simulink model "DepthTracking_ALOS_ADRC"  (R2020b)
settings: Solver=ode1  StartTime=0.0  StopTime=80  FixedStep=0.1  RelTol=1e-3
InitFcn:
  | InitParam;
undefined symbols (not defined in the file or in its folder): sigbuilder_block
settings Model: Creator=53549  LastModifiedBy=53549
settings DataIOCC: ReturnWorkspaceOutputs=off
settings DebuggingCC: ArithmeticOperatorsInVariantConditions=warning
settings SFSimCC: SimUseLocalCustomCode=off  CustomCodeUndefinedFunction=UseInterfaceOnly
settings RTWCC: RTWUseLocalCustomCode=off
settings CodeAppCC: StateflowObjectComments=on

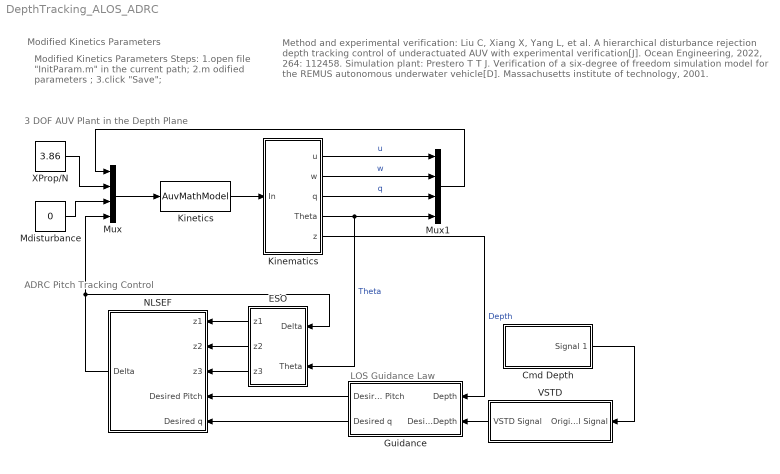
== system DepthTracking_ALOS_ADRC ==
  note: LOS Guidance Law
  note: ADRC Pitch Tracking Control
  note: 3 DOF AUV Plant in the Depth Plane
  note: Method and experimental verification: Liu C, Xiang X, Yang L, et al. A hierarchical disturbance rejection depth tracking control of underactuated AUV with experimental verification[J]. Ocean Engineering, 2022, 264: 112458.
      | Simulation plant: Prestero T T J. Verification of a six-degree of freedom simulation model for the REMUS autonomous underwater vehicle[D]. Massachusetts institute of technology, 2001.
  note: Modified Kinetics Parameters Steps:
      | 1.open file "InitParam.m" in the current path;
      | 2.m odified parameters ;
      | 3.click "Save";
  note: Modified Kinetics Parameters
  Cmd Depth : Subsystem  Tag=STV Subsys  LoadFcn=sigbuilder_block('load');  StartFcn=sigbuilder_block('start');  StopFcn=sigbuilder_block('stop');  ClipboardFcn=sigbuilder_block('clipboard');  mask(Sigbuilder block){tuvar=[0:10]}
      mask help: Simulink:masks:SigbuilderBlock_MD
      mask init:
      | if ~strcmp(get_param(bdroot(gcbh),'SimulationStatus'),'stopped') tuvar = sigbuilder_block('maskInit'); end
      settings: CopyFcn=sigbuilder_block('copy');  DeleteFcn=sigbuilder_block('delete');  ModelCloseFcn=sigbuilder_block('modelClose');  PreSaveFcn=sigbuilder_block('preSave');  PauseFcn=sigbuilder_block('pause');  ContinueFcn=sigbuilder_block('continue');  NameChangeFcn=sigbuilder_block('namechange');  OpenFcn=sigbuilder_block('open',[75 86 550.5 363 ]);  CloseFcn=sigbuilder_block('close');
      mask Display: plot(0, 0, 100, 100,[2, 2, 32, 32, 2], [68, 8, 8, 68, 68],[32, 2], [38, 38], [32, 19, 2],[53, 60, 44], [32, 17, 17, 2],[16, 16, 31, 31]);txt = getActiveGroup(gcbh);text(2, 100, txt,'verticalAlignment', 'top');
  ESO : Subsystem
  Guidance : Subsystem  mask{losAlg=ALOS, klos=3, KIlos=0.01}
      mask prompts: losAlg "LOS Form"; klos "Forward Distance"; KIlos "Integral gain"
      mask TypeOptions losAlg: LOS | ALOS
      mask DialogControl DescGroupVar Prompt: Guidance
      mask DialogControl DescTextVar Prompt: Select LOS or ALOS guidance algorithm and set parameters
      mask DialogControl ParameterGroupVar Prompt: LOS parameters
  Kinematics : Subsystem  mask{z0=0.2, u0=1.4, theta0=0}
      mask prompts: z0 "Initial Depth"; u0 "Initial Velocity"; theta0 "Initial Pitch[Deg]"
      mask DialogControl DescGroupVar Prompt: Initial Motion State
      mask DialogControl DescTextVar Prompt: Set initial state: depth, velocity, pitch
  Kinetics : MATLABFcn  MATLABFcn=AuvMathModel  OutputDimensions=4  OutputSignalType=real
  Mdisturbance : Constant  Value=0
  Mux : Mux
  Mux1 : Mux
  NLSEF : Subsystem  mask{FDForm=NLSEF, beta1=3, beta2=4, c=0.8, r=35, h=0.5, k1=0.07, k2=0.04}
      mask prompts: FDForm "NLSEF Form"; beta1 "β1"; beta2 "β2"
      mask TypeOptions FDForm: LSEF | NLSEF | S Surface
      mask DialogControl DescGroupVar Prompt: NLSEF
      mask DialogControl Control4 Prompt: Select the form of error feedback law and set corresponding parameters
      mask DialogControl ParameterGroupVar Prompt: NLSEF
      mask DialogControl Container3 Prompt: LSEF Parameter
      mask DialogControl Container4 Prompt: NLSEF Parameter
      mask DialogControl Container5 Prompt: S Surface Parameter
  VSTD : Subsystem  mask{InitValue=0.2, r=0.05, h=0.1}
      mask prompts: InitValue "InitSignalValue"
      mask DialogControl DescGroupVar Prompt: 最速跟踪微分器
  XProp/N : Constant  Value=3.86
  wires:
  Kinetics/1 -> Kinematics/1(In)
  Mux/1 -> Kinetics/1
  Kinematics/4(Theta) -> Mux1/4, ESO/2(Theta)  "Theta"
  Kinematics/1(u) -> Mux1/1  "u"
  Kinematics/2(w) -> Mux1/2  "w"
  Kinematics/3(q) -> Mux1/3  "q"
  Mux1/1 -> Mux/1
  XProp/N/1 -> Mux/2
  Kinematics/5(z) -> Guidance/1(Depth)  "Depth"
  Cmd Depth/1(Signal 1) -> VSTD/1(Original Signal)
  ESO/1(z1) -> NLSEF/1(z1)
  ESO/2(z2) -> NLSEF/2(z2)
  ESO/3(z3) -> NLSEF/3(z3)
  VSTD/1(VSTD Signal) -> Guidance/2(Desired Depth)
  Guidance/1(Desired Pitch) -> NLSEF/4(Desired Pitch)
  Mdisturbance/1 -> Mux/3
  NLSEF/1(Delta) -> Mux/4, ESO/1(Delta)
  Guidance/2("Desired q  ") -> NLSEF/5("Desired q ")

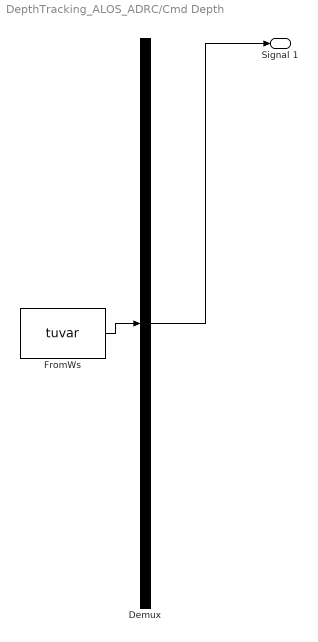
== system DepthTracking_ALOS_ADRC/Cmd Depth ==
  Demux : Demux  Tag=STV Demux  Outputs=1
      settings: DisplayOption=none
  FromWs : FromWorkspace  Tag=STV FromWs  VariableName=tuvar
      SigBuilderData=|
      | common.afterFinalStr = 'Extrapolate'
      | common.sampleTime = 0
      | dataSet.timeRange = [0 80]
      | dataSet.name = 'Group 1'
      | sbobj.Groups.Name = 'Group 1'
      | sbobj.Groups.Signals.Name = 'Signal 1'
      | sbobj.Groups.Signals.XData = [0 4 60 60 80]
      | sbobj.Groups.Signals.YData = [3 3 3 0 0]
      | sbobj.Groups.TimeRange = [0 80]
  Signal 1 : Outport  Tag=STV Outport
  wires:
  Demux/1 -> Signal 1/1
  FromWs/1 -> Demux/1

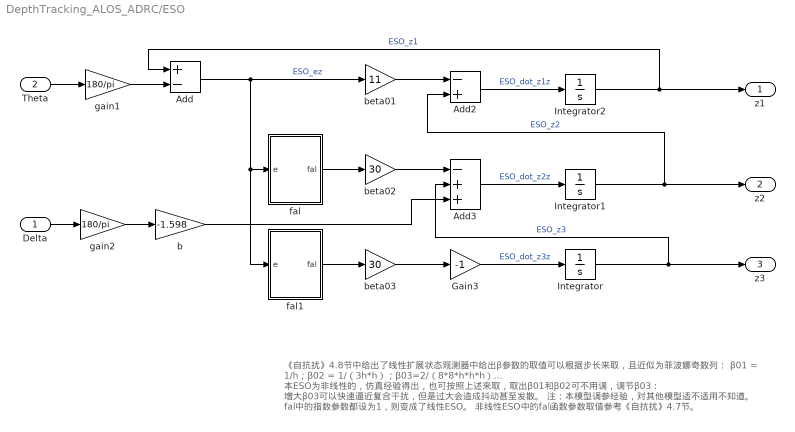
== system DepthTracking_ALOS_ADRC/ESO ==
  note: 《自抗扰》4.8节中给出了线性扩展状态观测器中给出β参数的取值可以根据步长来取，且近似为菲波娜奇数列：
      | β01 = 1/h；β02 = 1/（3h*h）；β03=2/（8*8*h*h*h）...
      | 本ESO为非线性的，仿真经验得出，也可按照上述来取，取出β01和β02可不用调，调节β03：
      | 增大β03可以快速逼近复合干扰，但是过大会造成抖动甚至发散。
      | 注：本模型调参经验，对其他模型适不适用不知道。
      | fal中的指数参数都设为1，则变成了线性ESO。
      | 非线性ESO中的fal函数参数取值参考《自抗扰》4.7节。
  Delta : Inport
  Theta : Inport  Port=2
  Add : Sum  Inputs=+-
  Add2 : Sum  Inputs=-+
  Add3 : Sum  Inputs=-++
  Gain3 : Gain  Gain=-1
  Integrator : Integrator
  Integrator1 : Integrator
  Integrator2 : Integrator
  b : Gain  Gain=-1.598
  beta01 : Gain  Gain=11
  beta02 : Gain  Gain=30
  beta03 : Gain  Gain=30
  fal : Subsystem  mask{a=0.5, sat=0.1}
      mask prompts: a "指数"; sat "边界"
      mask help: fal函数
      mask Display: disp('fal(e,a,sat)');
  fal1 : Subsystem  mask{a=0.25, sat=0.1}
      mask prompts: a "指数"; sat "边界"
      mask help: fal函数
      mask Display: disp('fal(e,a,sat)');
  gain1 : Gain  Gain=180/pi
  gain2 : Gain  Gain=180/pi
  z1 : Outport
  z2 : Outport  Port=2
  z3 : Outport  Port=3
  wires:
  Integrator2/1 -> Add/1, z1/1  "ESO_z1"
  Gain3/1 -> Integrator/1  "ESO_dot_z3z"
  beta03/1 -> Gain3/1
  fal1/1(fal) -> beta03/1
  Add3/1 -> Integrator1/1  "ESO_dot_z2z"
  Integrator/1 -> Add3/2, z3/1  "ESO_z3"
  beta02/1 -> Add3/1
  fal/1(fal) -> beta02/1
  Add2/1 -> Integrator2/1  "ESO_dot_z1z"
  Integrator1/1 -> Add2/2, z2/1  "ESO_z2"
  beta01/1 -> Add2/1
  Add/1 -> beta01/1, fal/1(e), fal1/1(e)  "ESO_ez"
  Theta/1 -> gain1/1
  Delta/1 -> gain2/1
  b/1 -> Add3/3
  gain1/1 -> Add/2
  gain2/1 -> b/1

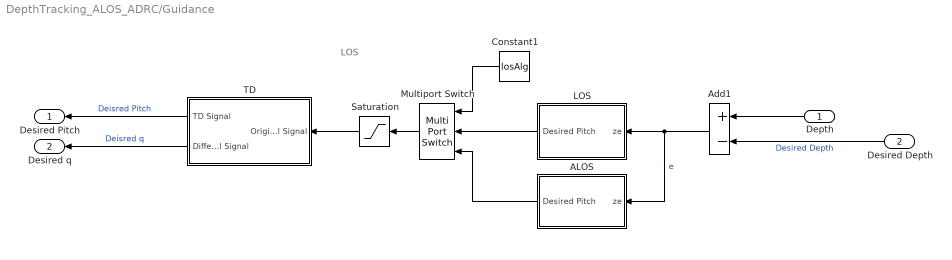
== system DepthTracking_ALOS_ADRC/Guidance ==
  note: LOS
  Depth : Inport
  Desired Depth : Inport  Port=2
  ALOS : Subsystem
  Add1 : Sum  Inputs=+-
  Constant1 : Constant  Value=losAlg
  LOS : Subsystem
  Multiport Switch : MultiPortSwitch  Inputs=2
  Saturation : Saturate  UpperLimit=25  LowerLimit=-25
  TD : Subsystem  mask{InitValue=0, r=10, h=0.1}
      mask prompts: InitValue "InitSignalValue"
      mask DialogControl DescGroupVar Prompt: 最速跟踪微分器
  Desired Pitch : Outport
  "Desired q  " : Outport  Port=2
  wires:
  Desired Depth/1 -> Add1/2  "Desired Depth"
  Saturation/1 -> TD/1(Original Signal)
  Multiport Switch/1 -> Saturation/1
  TD/1(TD Signal) -> Desired Pitch/1  "Deisred Pitch"
  TD/2(Differential Signal) -> "Desired q  "/1  "Deisred q"
  LOS/1(Desired Pitch) -> Multiport Switch/2
  ALOS/1(Desired Pitch) -> Multiport Switch/3
  Add1/1 -> ALOS/1(ze), LOS/1(ze)  "e"
  Constant1/1 -> Multiport Switch/1
  Depth/1 -> Add1/1

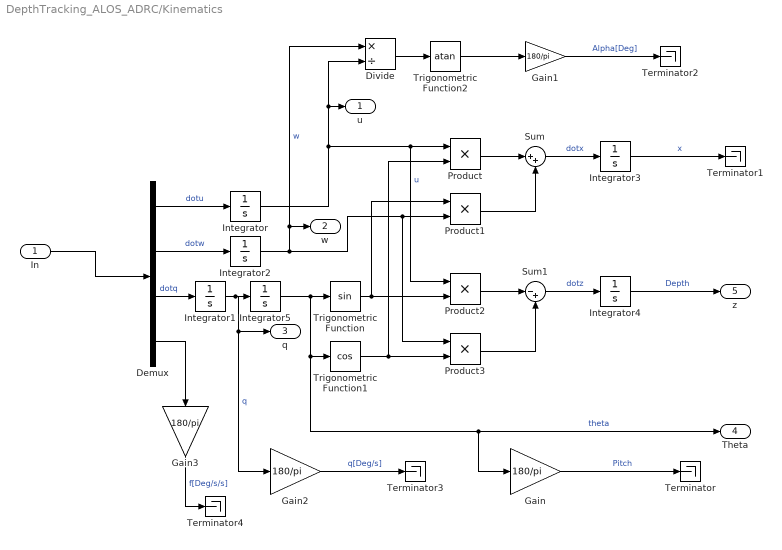
== system DepthTracking_ALOS_ADRC/Kinematics ==
  In : Inport
  Demux : Demux
  Divide : Product  Inputs=*/
  Gain{,1..3} (4 alike) : Gain  Gain=180/pi
  Integrator : Integrator  InitialCondition=u0  ContinuousStateAttributes='u'
  Integrator1 : Integrator  ContinuousStateAttributes='q'
  Integrator2 : Integrator  ContinuousStateAttributes='w'
  Integrator3 : Integrator
  Integrator4 : Integrator  InitialCondition=z0
  Integrator5 : Integrator  InitialCondition=theta0/180*pi  ContinuousStateAttributes='theta'
  Product{,1..3} (4 alike) : Product
  Sum : Sum  Inputs=|++
  Sum1 : Sum  Inputs=|-+
  Terminator{,1..4} (5 alike) : Terminator
  Trigonometric Function : Trigonometry
  Trigonometric Function1 : Trigonometry  Operator=cos
  Trigonometric Function2 : Trigonometry  Operator=atan
  u : Outport
  w : Outport  Port=2
  q : Outport  Port=3
  Theta : Outport  Port=4
  z : Outport  Port=5
  wires:
  Integrator3/1 -> Terminator1/1  "x"
  Product2/1 -> Sum1/1
  Product1/1 -> Sum/2
  Demux/1 -> Integrator/1  "dotu"
  Demux/2 -> Integrator2/1  "dotw"
  Demux/3 -> Integrator1/1  "dotq"
  Trigonometric Function1/1 -> Product/2, Product3/2
  Product/1 -> Sum/1
  Product3/1 -> Sum1/2
  In/1 -> Demux/1
  Integrator4/1 -> z/1  "Depth"
  Sum/1 -> Integrator3/1  "dotx"
  Trigonometric Function/1 -> Product1/1, Product2/2
  Sum1/1 -> Integrator4/1  "dotz"
  Integrator1/1 -> Gain2/1, q/1, Integrator5/1  "q"
  Integrator5/1 -> Gain/1, Theta/1, Trigonometric Function1/1, Trigonometric Function/1  "theta"
  Gain/1 -> Terminator/1  "Pitch"
  Trigonometric Function2/1 -> Gain1/1
  Divide/1 -> Trigonometric Function2/1
  Integrator2/1 -> Divide/1, w/1, Product1/2, Product3/1  "w"
  Integrator/1 -> Divide/2, u/1, Product/1, Product2/1  "u"
  Gain1/1 -> Terminator2/1  "Alpha[Deg]"
  Gain2/1 -> Terminator3/1  "q[Deg/s]"
  Demux/4 -> Gain3/1
  Gain3/1 -> Terminator4/1  "f[Deg/s/s]"

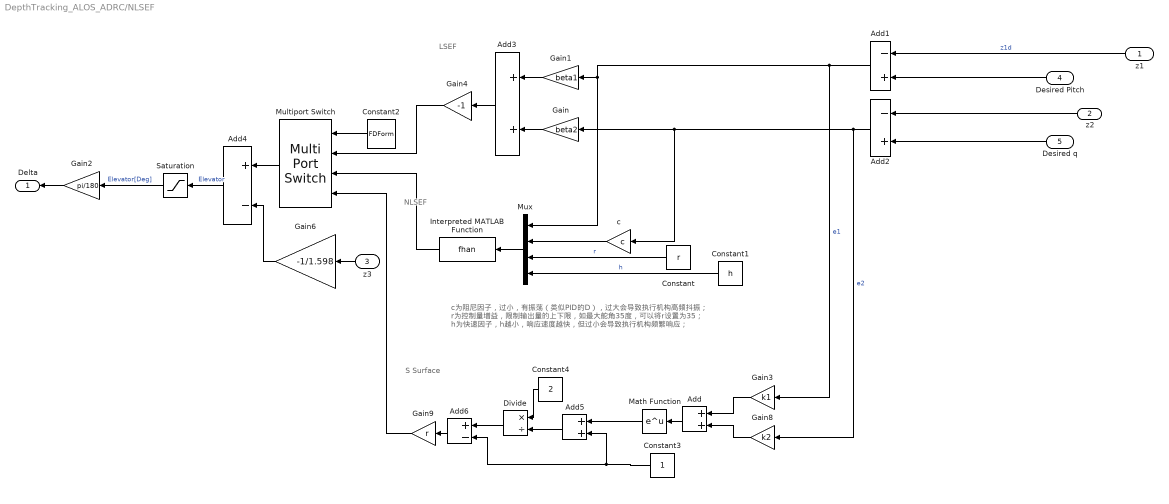
== system DepthTracking_ALOS_ADRC/NLSEF ==
  note: S Surface
  note: NLSEF
  note: LSEF
  note: c为阻尼因子，过小，有振荡（类似PID的D），过大会导致执行机构高频抖振；
      | r为控制量增益，限制输出量的上下限，如最大舵角35度，可以将r设置为35；
      | h为快速因子，h越小，响应速度越快，但过小会导致执行机构频繁响应；
  z1 : Inport
  z2 : Inport  Port=2
  z3 : Inport  Port=3
  Desired Pitch : Inport  Port=4
  "Desired q " : Inport  Port=5
  Add : Sum
  Add1 : Sum  Inputs=-+
  Add2 : Sum  Inputs=-+
  Add3 : Sum
  Add4 : Sum  Inputs=+-
  Add5 : Sum
  Add6 : Sum  Inputs=+-
  Constant : Constant  Value=r
  Constant1 : Constant  Value=h
  Constant2 : Constant  Value=FDForm
  Constant3 : Constant
  Constant4 : Constant  Value=2
  Divide : Product  Inputs=*/
  Gain : Gain  Gain=beta2
  Gain1 : Gain  Gain=beta1
  Gain2 : Gain  Gain=pi/180
  Gain3 : Gain  Gain=k1
  Gain4 : Gain  Gain=-1
  Gain6 : Gain  Gain=-1/1.598
  Gain8 : Gain  Gain=k2
  Gain9 : Gain  Gain=r
  Interpreted MATLAB Function : MATLABFcn  MATLABFcn=fhan  OutputDimensions=1
  Math Function : Math  SaturateOnIntegerOverflow=on
  Multiport Switch : MultiPortSwitch
  Mux : Mux
  Saturation : Saturate  UpperLimit=35  LowerLimit=-35
  c : Gain  Gain=c
  Delta : Outport
  wires:
  Add1/1 -> Gain3/1, Gain1/1, Mux/1  "e1"
  Desired Pitch/1 -> Add1/2
  "Desired q "/1 -> Add2/2
  Add2/1 -> Gain8/1, Gain/1, c/1  "e2"
  Gain2/1 -> Delta/1
  Gain/1 -> Add3/2
  Gain1/1 -> Add3/1
  z1/1 -> Add1/1  "z1d"
  Multiport Switch/1 -> Add4/1
  Add3/1 -> Gain4/1
  Mux/1 -> Interpreted MATLAB Function/1
  c/1 -> Mux/2
  Constant/1 -> Mux/3  "r"
  Gain4/1 -> Multiport Switch/2
  Interpreted MATLAB Function/1 -> Multiport Switch/3
  Constant1/1 -> Mux/4  "h"
  Add4/1 -> Saturation/1  "Elevator"
  z3/1 -> Gain6/1
  Constant2/1 -> Multiport Switch/1
  z2/1 -> Add2/1
  Gain3/1 -> Add/1
  Gain8/1 -> Add/2
  Add/1 -> Math Function/1
  Math Function/1 -> Add5/1
  Constant3/1 -> Add6/2, Add5/2
  Add5/1 -> Divide/2
  Constant4/1 -> Divide/1
  Divide/1 -> Add6/1
  Gain9/1 -> Multiport Switch/4
  Add6/1 -> Gain9/1
  Gain6/1 -> Add4/2
  Saturation/1 -> Gain2/1  "Elevator[Deg]"

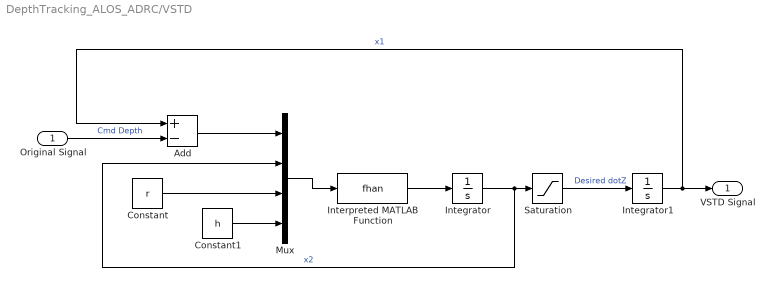
== system DepthTracking_ALOS_ADRC/VSTD ==
  Original Signal : Inport
  Add : Sum  Inputs=+-
  Constant : Constant  Value=r
  Constant1 : Constant  Value=h
  Integrator : Integrator
  Integrator1 : Integrator  InitialCondition=InitValue
  Interpreted MATLAB Function : MATLABFcn  MATLABFcn=fhan  OutputDimensions=1
  Mux : Mux
  Saturation : Saturate  UpperLimit=0.2  LowerLimit=-0.2
  VSTD Signal : Outport
  wires:
  Add/1 -> Mux/1
  Constant/1 -> Mux/3
  Constant1/1 -> Mux/4
  Mux/1 -> Interpreted MATLAB Function/1
  Interpreted MATLAB Function/1 -> Integrator/1
  Integrator/1 -> Saturation/1, Mux/2  "x2"
  Integrator1/1 -> Add/1, VSTD Signal/1  "x1"
  Original Signal/1 -> Add/2  "Cmd Depth"
  Saturation/1 -> Integrator1/1  "Desired dotZ"

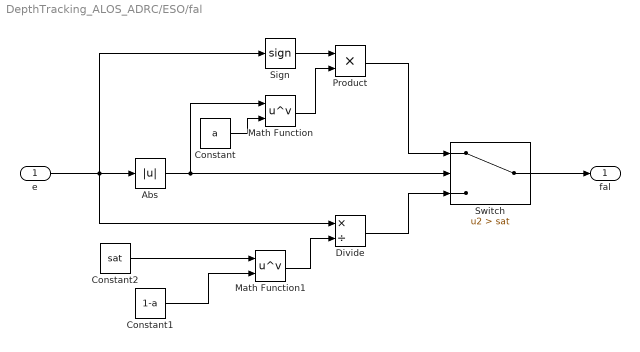
== system DepthTracking_ALOS_ADRC/ESO/fal ==
  e : Inport
  Abs : Abs
  Constant : Constant  Value=a
  Constant1 : Constant  Value=1-a
  Constant2 : Constant  Value=sat
  Divide : Product  Inputs=*/
  Math Function : Math  Operator=pow  SignedPower=on  SaturateOnIntegerOverflow=on
  Math Function1 : Math  Operator=pow  SignedPower=on  SaturateOnIntegerOverflow=on
  Product : Product
  Sign : Signum
  Switch : Switch  Criteria=u2 > Threshold  Threshold=sat
  fal : Outport
  wires:
  Constant2/1 -> Math Function1/1
  Constant/1 -> Math Function/2
  Math Function/1 -> Product/2
  Divide/1 -> Switch/3
  Math Function1/1 -> Divide/2
  Switch/1 -> fal/1
  Product/1 -> Switch/1
  Sign/1 -> Product/1
  Abs/1 -> Switch/2, Math Function/1
  Constant1/1 -> Math Function1/2
  e/1 -> Abs/1, Sign/1, Divide/1

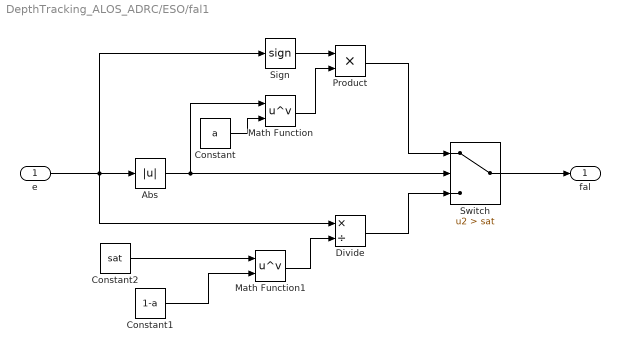
== system DepthTracking_ALOS_ADRC/ESO/fal1 ==
  e : Inport
  Abs : Abs
  Constant : Constant  Value=a
  Constant1 : Constant  Value=1-a
  Constant2 : Constant  Value=sat
  Divide : Product  Inputs=*/
  Math Function : Math  Operator=pow  SignedPower=on  SaturateOnIntegerOverflow=on
  Math Function1 : Math  Operator=pow  SignedPower=on  SaturateOnIntegerOverflow=on
  Product : Product
  Sign : Signum
  Switch : Switch  Criteria=u2 > Threshold  Threshold=sat
  fal : Outport
  wires:
  e/1 -> Divide/1, Sign/1, Abs/1
  Constant1/1 -> Math Function1/2
  Abs/1 -> Math Function/1, Switch/2
  Sign/1 -> Product/1
  Product/1 -> Switch/1
  Switch/1 -> fal/1
  Math Function1/1 -> Divide/2
  Divide/1 -> Switch/3
  Math Function/1 -> Product/2
  Constant/1 -> Math Function/2
  Constant2/1 -> Math Function1/1

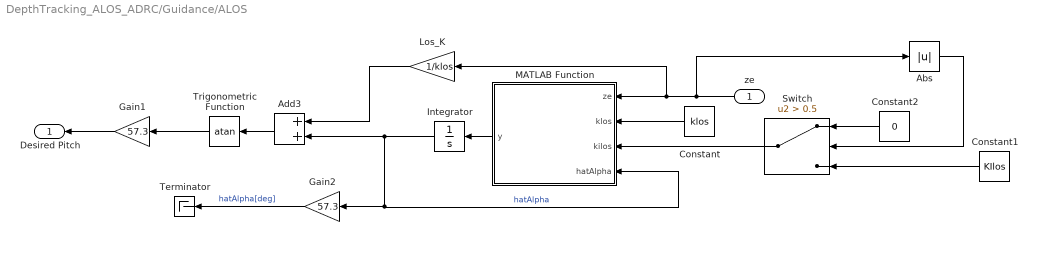
== system DepthTracking_ALOS_ADRC/Guidance/ALOS ==
  ze : Inport
  Abs : Abs
  Add3 : Sum
  Constant : Constant  Value=klos
  Constant1 : Constant  Value=KIlos
  Constant2 : Constant  Value=0
  Gain1 : Gain  Gain=57.3
  Gain2 : Gain  Gain=57.3
  Integrator : Integrator
  Los_K : Gain  Gain=1/klos
  MATLAB Function : MATLAB Function  TreatAsAtomicUnit=on
  Switch : Switch  Criteria=u2 > Threshold  Threshold=0.5
  Terminator : Terminator
  Trigonometric Function : Trigonometry  Operator=atan
  Desired Pitch : Outport
  wires:
  Integrator/1 -> MATLAB Function/4(hatAlpha), Gain2/1, Add3/2  "hatAlpha"
  Constant/1 -> MATLAB Function/2(klos)
  MATLAB Function/1(y) -> Integrator/1
  ze/1 -> Abs/1, Los_K/1, MATLAB Function/1(ze)
  Los_K/1 -> Add3/1
  Add3/1 -> Trigonometric Function/1
  Gain1/1 -> Desired Pitch/1
  Trigonometric Function/1 -> Gain1/1
  Gain2/1 -> Terminator/1  "hatAlpha[deg]"
  Switch/1 -> MATLAB Function/3(kilos)
  Constant1/1 -> Switch/3
  Abs/1 -> Switch/2
  Constant2/1 -> Switch/1

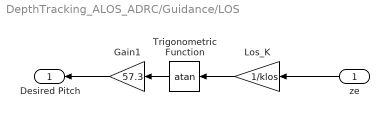
== system DepthTracking_ALOS_ADRC/Guidance/LOS ==
  ze : Inport
  Gain1 : Gain  Gain=57.3
  Los_K : Gain  Gain=1/klos
  Trigonometric Function : Trigonometry  Operator=atan
  Desired Pitch : Outport
  wires:
  Los_K/1 -> Trigonometric Function/1
  Trigonometric Function/1 -> Gain1/1
  ze/1 -> Los_K/1
  Gain1/1 -> Desired Pitch/1

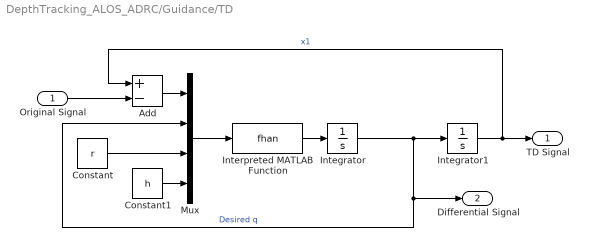
== system DepthTracking_ALOS_ADRC/Guidance/TD ==
  Original Signal : Inport
  Add : Sum  Inputs=+-
  Constant : Constant  Value=r
  Constant1 : Constant  Value=h
  Integrator : Integrator
  Integrator1 : Integrator  InitialCondition=InitValue
  Interpreted MATLAB Function : MATLABFcn  MATLABFcn=fhan  OutputDimensions=1
  Mux : Mux
  TD Signal : Outport
  Differential Signal : Outport  Port=2
  wires:
  Add/1 -> Mux/1
  Constant/1 -> Mux/3
  Constant1/1 -> Mux/4
  Mux/1 -> Interpreted MATLAB Function/1
  Interpreted MATLAB Function/1 -> Integrator/1
  Integrator/1 -> Integrator1/1, Mux/2, Differential Signal/1  "Desired q"
  Integrator1/1 -> TD Signal/1, Add/1  "x1"
  Original Signal/1 -> Add/2

== matlab function DepthTracking_ALOS_ADRC/Guidance/ALOS/MATLAB Function ==
  data: ze input; y output; klos input; kilos input; hatAlpha input
function y = fcn(ze,klos,kilos,hatAlpha)
y =1.45*ze*klos*kilos/sqrt(klos*klos+(ze+klos*hatAlpha)*(ze+klos*hatAlpha));
